simulink model "canPack_ADC1_EPS_01"  (R2020a)
settings: Solver=VariableStepAuto  StartTime=0.0  StopTime=10.0  RelTol=1e-3
libraries: MyLibrary x1
settings Model: Creator=Administrator  LastModifiedBy=Administrator

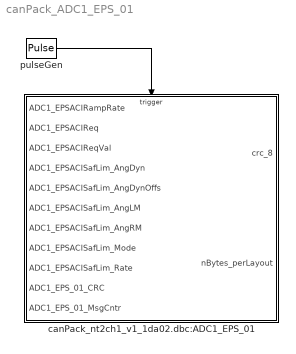
== system canPack_ADC1_EPS_01 ==
  canPack_nt2ch1_v1_1da02.dbc:ADC1_EPS_01 : Subsystem
  pulseGen : DiscretePulseGenerator  PulseType=Time based  Period=0.02  PulseWidth=50
  wires:
  pulseGen/1 -> canPack_nt2ch1_v1_1da02.dbc:ADC1_EPS_01/Trigger

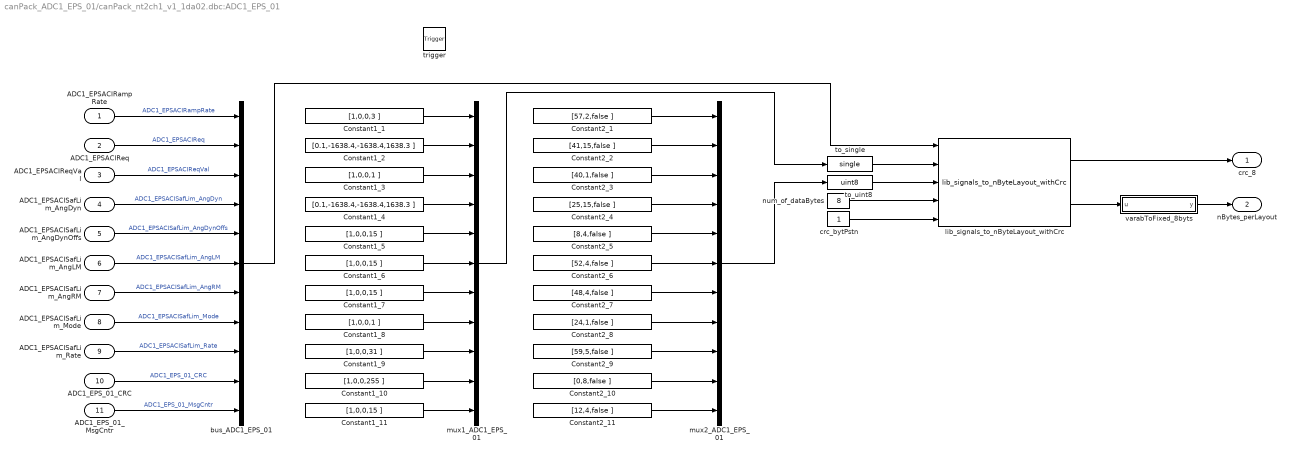
== system canPack_ADC1_EPS_01/canPack_nt2ch1_v1_1da02.dbc:ADC1_EPS_01 ==
  ADC1_EPSACIRampRate : Inport
  ADC1_EPSACIReq : Inport  Port=2
  ADC1_EPSACIReqVal : Inport  Port=3
  ADC1_EPSACISafLim_AngDyn : Inport  Port=4
  ADC1_EPSACISafLim_AngDynOffs : Inport  Port=5
  ADC1_EPSACISafLim_AngLM : Inport  Port=6
  ADC1_EPSACISafLim_AngRM : Inport  Port=7
  ADC1_EPSACISafLim_Mode : Inport  Port=8
  ADC1_EPSACISafLim_Rate : Inport  Port=9
  ADC1_EPS_01_CRC : Inport  Port=10
  ADC1_EPS_01_MsgCntr : Inport  Port=11
  trigger : TriggerPort  VariantControl=Variant  PortDimensions=1
  Constant1_1 : Constant  Value=[1,0,0,3 ]  SampleTime=-1
  Constant1_10 : Constant  Value=[1,0,0,255 ]  SampleTime=-1
  Constant1_{5..7,11} (4 alike) : Constant  Value=[1,0,0,15 ]  SampleTime=-1
  Constant1_2 : Constant  Value=[0.1,-1638.4,-1638.4,1638.3 ]  SampleTime=-1
  Constant1_3 : Constant  Value=[1,0,0,1 ]  SampleTime=-1
  Constant1_4 : Constant  Value=[0.1,-1638.4,-1638.4,1638.3 ]  SampleTime=-1
  Constant1_8 : Constant  Value=[1,0,0,1 ]  SampleTime=-1
  Constant1_9 : Constant  Value=[1,0,0,31 ]  SampleTime=-1
  Constant2_1 : Constant  Value=[57,2,false ]  SampleTime=-1
  Constant2_10 : Constant  Value=[0,8,false ]  SampleTime=-1
  Constant2_11 : Constant  Value=[12,4,false ]  SampleTime=-1
  Constant2_2 : Constant  Value=[41,15,false ]  SampleTime=-1
  Constant2_3 : Constant  Value=[40,1,false ]  SampleTime=-1
  Constant2_4 : Constant  Value=[25,15,false ]  SampleTime=-1
  Constant2_5 : Constant  Value=[8,4,false ]  SampleTime=-1
  Constant2_6 : Constant  Value=[52,4,false ]  SampleTime=-1
  Constant2_7 : Constant  Value=[48,4,false ]  SampleTime=-1
  Constant2_8 : Constant  Value=[24,1,false ]  SampleTime=-1
  Constant2_9 : Constant  Value=[59,5,false ]  SampleTime=-1
  bus_ADC1_EPS_01 : BusCreator  Inputs=11
  crc_bytPstn : Constant  OutDataTypeStr=uint8  SampleTime=-1
  lib_signals_to_nByteLayout_withCrc : MyLibrary/lib_signals_to_nByteLayout_withCrc  SystemSampleTime=-1  Latency=0  AutoFrameSizeCalculation=off
  mux1_ADC1_EPS_01 : Mux  Inputs=11
  mux2_ADC1_EPS_01 : Mux  Inputs=11
  num_of_dataBytes : Constant  Value=8  OutDataTypeStr=uint8  SampleTime=-1
  to_single : DataTypeConversion  OutDataTypeStr=single
  to_uint8 : DataTypeConversion  OutDataTypeStr=uint8
  varabToFixed_8byts : MATLAB Function  TreatAsAtomicUnit=on
  crc_8 : Outport
  nBytes_perLayout : Outport  Port=2
  wires:
  ADC1_EPSACIRampRate/1 -> bus_ADC1_EPS_01/1  "ADC1_EPSACIRampRate"
  ADC1_EPSACIReq/1 -> bus_ADC1_EPS_01/2  "ADC1_EPSACIReq"
  ADC1_EPSACIReqVal/1 -> bus_ADC1_EPS_01/3  "ADC1_EPSACIReqVal"
  ADC1_EPSACISafLim_AngDyn/1 -> bus_ADC1_EPS_01/4  "ADC1_EPSACISafLim_AngDyn"
  ADC1_EPSACISafLim_AngDynOffs/1 -> bus_ADC1_EPS_01/5  "ADC1_EPSACISafLim_AngDynOffs"
  ADC1_EPSACISafLim_AngLM/1 -> bus_ADC1_EPS_01/6  "ADC1_EPSACISafLim_AngLM"
  ADC1_EPSACISafLim_AngRM/1 -> bus_ADC1_EPS_01/7  "ADC1_EPSACISafLim_AngRM"
  ADC1_EPSACISafLim_Mode/1 -> bus_ADC1_EPS_01/8  "ADC1_EPSACISafLim_Mode"
  ADC1_EPSACISafLim_Rate/1 -> bus_ADC1_EPS_01/9  "ADC1_EPSACISafLim_Rate"
  ADC1_EPS_01_CRC/1 -> bus_ADC1_EPS_01/10  "ADC1_EPS_01_CRC"
  ADC1_EPS_01_MsgCntr/1 -> bus_ADC1_EPS_01/11  "ADC1_EPS_01_MsgCntr"
  Constant1_1/1 -> mux1_ADC1_EPS_01/1
  Constant2_1/1 -> mux2_ADC1_EPS_01/1
  Constant1_2/1 -> mux1_ADC1_EPS_01/2
  Constant2_2/1 -> mux2_ADC1_EPS_01/2
  Constant1_3/1 -> mux1_ADC1_EPS_01/3
  Constant2_3/1 -> mux2_ADC1_EPS_01/3
  Constant1_4/1 -> mux1_ADC1_EPS_01/4
  Constant2_4/1 -> mux2_ADC1_EPS_01/4
  Constant1_5/1 -> mux1_ADC1_EPS_01/5
  Constant2_5/1 -> mux2_ADC1_EPS_01/5
  Constant1_6/1 -> mux1_ADC1_EPS_01/6
  Constant2_6/1 -> mux2_ADC1_EPS_01/6
  Constant1_7/1 -> mux1_ADC1_EPS_01/7
  Constant2_7/1 -> mux2_ADC1_EPS_01/7
  Constant1_8/1 -> mux1_ADC1_EPS_01/8
  Constant2_8/1 -> mux2_ADC1_EPS_01/8
  Constant1_9/1 -> mux1_ADC1_EPS_01/9
  Constant2_9/1 -> mux2_ADC1_EPS_01/9
  Constant1_10/1 -> mux1_ADC1_EPS_01/10
  Constant2_10/1 -> mux2_ADC1_EPS_01/10
  Constant1_11/1 -> mux1_ADC1_EPS_01/11
  Constant2_11/1 -> mux2_ADC1_EPS_01/11
  bus_ADC1_EPS_01/1 -> lib_signals_to_nByteLayout_withCrc/1
  mux1_ADC1_EPS_01/1 -> to_single/1
  to_single/1 -> lib_signals_to_nByteLayout_withCrc/2
  mux2_ADC1_EPS_01/1 -> to_uint8/1
  to_uint8/1 -> lib_signals_to_nByteLayout_withCrc/3
  lib_signals_to_nByteLayout_withCrc/1 -> crc_8/1
  num_of_dataBytes/1 -> lib_signals_to_nByteLayout_withCrc/4
  lib_signals_to_nByteLayout_withCrc/2 -> varabToFixed_8byts/1(u)
  varabToFixed_8byts/1(y) -> nBytes_perLayout/1
  crc_bytPstn/1 -> lib_signals_to_nByteLayout_withCrc/5

== matlab function canPack_ADC1_EPS_01/canPack_nt2ch1_v1_1da02.dbc:ADC1_EPS_01/varabToFixed_8byts ==
  data: u input uint8 size=8; y output uint8
function y = fcn(u)

fixed_size = 8;
y = uint8(zeros(fixed_size,1));

for i=1:fixed_size
    y(i) = u(i);
end
